simulink model "ill_lf_1"  (R2018a)
settings: Solver=FixedStepAuto  StartTime=0.0  StopTime=10.0  RelTol=1e-3
libraries: arduinolib x10
settings Model: Creator=Admin  LastModifiedBy=DINESH

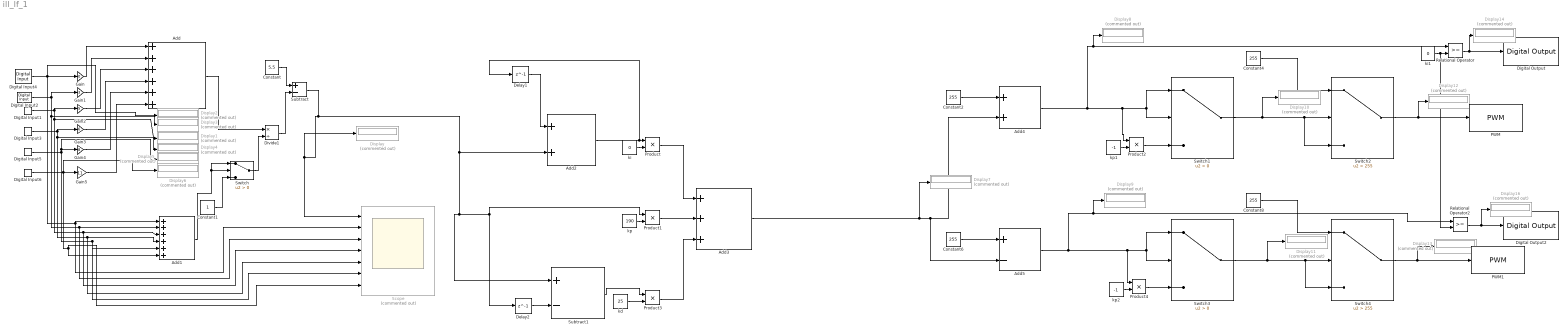
== system ill_lf_1 ==
  Add : Sum  Inputs=++++++
  Add1 : Sum  Inputs=++++++
  Add2 : Sum
  Add3 : Sum  Inputs=+++
  Add4 : Sum
  Add5 : Sum  Inputs=+-
  Constant : Constant  Value=5.5
  Constant1 : Constant
  Constant{2,4,6,8} (4 alike) : Constant  Value=255
  Delay1 : Delay  DelayLength=1  InitialCondition=0  SampleTime=0.001
  Delay2 : Delay  DelayLength=1  InitialCondition=0  SampleTime=0.001
  Digital Input1 : arduinolib/Digital Input  pinNumber=35  sampleTime=0.001  blockPlatform=arduino
      link override Digital Input: SampleTime=0.001
      settings: SourceProductName=Simulink Support Package for Arduino Hardware
  Digital Input2 : arduinolib/Digital Input  pinNumber=33  sampleTime=0.001  blockPlatform=arduino
      settings: SourceProductName=Simulink Support Package for Arduino Hardware
  Digital Input3 : arduinolib/Digital Input  pinNumber=37  sampleTime=0.001  blockPlatform=arduino
      settings: SourceProductName=Simulink Support Package for Arduino Hardware
  Digital Input4 : arduinolib/Digital Input  pinNumber=31  sampleTime=0.001  blockPlatform=arduino
      settings: SourceProductName=Simulink Support Package for Arduino Hardware
  Digital Input5 : arduinolib/Digital Input  pinNumber=39  sampleTime=0.001  blockPlatform=arduino
      settings: SourceProductName=Simulink Support Package for Arduino Hardware
  Digital Input6 : arduinolib/Digital Input  pinNumber=41  sampleTime=0.001  blockPlatform=arduino
      settings: SourceProductName=Simulink Support Package for Arduino Hardware
  Digital Output : arduinolib/Digital Output  pinNumber=13  blockPlatform=arduino
  Digital Output2 : arduinolib/Digital Output  pinNumber=12  blockPlatform=arduino
  Display{,1..14,16} (16 alike) : Display  Commented=on
  Divide1 : Product  Inputs=*/
  Gain : Gain  Gain=0
  Gain1 : Gain  Gain=3
  Gain2 : Gain  Gain=5
  Gain3 : Gain  Gain=6
  Gain4 : Gain  Gain=8
  Gain5 : Gain  Gain=11
  PWM : arduinolib/PWM  pinNumber=11  EnableInputFrequency=off  InitialFrequency=2000  InitialDutyCycle=0  NotificationType=None  blockPlatform=arduino
  PWM1 : arduinolib/PWM  pinNumber=3  EnableInputFrequency=off  InitialFrequency=2000  InitialDutyCycle=0  NotificationType=None  blockPlatform=arduino
  Product{,1..4} (5 alike) : Product
  Relational Operator : RelationalOperator  OutDataTypeStr=boolean  RndMeth=Simplest
  Relational Operator2 : RelationalOperator  OutDataTypeStr=boolean  RndMeth=Simplest
  Scope : Scope  Commented=on  NumInputPorts=7
  Subtract : Sum  Inputs=+-
  Subtract1 : Sum  Inputs=+-
  Switch : Switch  Criteria=u2 > Threshold
  Switch1 : Switch  Criteria=u2 > Threshold
  Switch2 : Switch  Criteria=u2 > Threshold  Threshold=255
  Switch3 : Switch  Criteria=u2 > Threshold
  Switch4 : Switch  Criteria=u2 > Threshold  Threshold=255
  kd : Constant  Value=25
  ki : Constant  Value=0
  ki1 : Constant  Value=0
  kp : Constant  Value=190
  kp1 : Constant  Value=-1
  kp2 : Constant  Value=-1
  wires:
  Constant1/1 -> Switch/3
  kd/1 -> Product3/2
  Divide1/1 -> Subtract/2
  Constant/1 -> Subtract/1
  Gain5/1 -> Add/6
  Relational Operator/1 -> Display14/1, Digital Output/1
  Gain4/1 -> Add/5
  Subtract1/1 -> Product3/1
  Product1/1 -> Add3/2
  Digital Input2/1 -> Gain1/1, Display3/1, Scope/3, Add1/2
  Delay2/1 -> Subtract1/2
  Switch1/1 -> Display10/1, Switch2/3, Switch2/2
  Constant6/1 -> Add5/1
  Digital Input6/1 -> Scope/7, Add1/6, Display6/1, Gain5/1
  Add2/1 -> Delay1/1, Product/1
  Gain3/1 -> Add/4
  Product/1 -> Add3/1
  Digital Input3/1 -> Gain3/1, Display4/1, Scope/5, Add1/4
  Add1/1 -> Switch/1, Switch/2
  Constant2/1 -> Add4/1
  Add4/1 -> Display8/1, Relational Operator/1, Product2/1, Switch1/2, Switch1/1
  Digital Input1/1 -> Gain2/1, Display1/1, Scope/4, Add1/3
  Digital Input5/1 -> Display5/1, Gain4/1, Scope/6, Add1/5
  Digital Input4/1 -> Display2/1, Scope/2, Add1/1, Gain/1
  Constant8/1 -> Switch4/1
  Switch2/1 -> Display12/1, PWM/1
  Add5/1 -> Display9/1, Relational Operator2/1, Product4/1, Switch3/1, Switch3/2
  Switch4/1 -> Display13/1, PWM1/1
  Product3/1 -> Add3/3
  kp/1 -> Product1/2
  Constant4/1 -> Switch2/1
  Delay1/1 -> Add2/1
  Product4/1 -> Switch3/3
  Switch/1 -> Divide1/2
  ki/1 -> Product/2
  Gain2/1 -> Add/3
  kp1/1 -> Product2/2
  Add/1 -> Divide1/1
  Product2/1 -> Switch1/3
  Relational Operator2/1 -> Display16/1, Digital Output2/1
  Switch3/1 -> Display11/1, Switch4/3, Switch4/2
  Gain1/1 -> Add/2
  Gain/1 -> Add/1
  ki1/1 -> Relational Operator2/2, Relational Operator/2
  Add3/1 -> Display7/1, Add5/2, Add4/2
  kp2/1 -> Product4/2
  Subtract/1 -> Scope/1, Display/1, Subtract1/1, Product1/1, Delay2/1, Add2/2
